simulink model "AttitudeControl_ADRC_Sim"  (R2017b)
settings: Solver=ode4  StartTime=0.0  StopTime=2  FixedStep=0.004  RelTol=1e-3
StartFcn:
  | Init_control_adrc
values from neighbouring files (symbols this model uses):
  DEG2RAD = 0.0174533    [Init_control_adrc.m]
  DisturbOn = 0    [Init_control_adrc.m]
  Kd_YAW_AngleRate = 0.00    (= 0)    [Init_control_adrc.m]
  Ki_YAW_AngleRate = 0.01    [Init_control_adrc.m]
  Kp_YAW_AngleRate = 0.5    [Init_control_adrc.m]
  MAX_CONTROL_ANGLE_PITCH = 35    [Init_control_adrc.m]
  MAX_CONTROL_ANGLE_RATE_Y = 200    [Init_control_adrc.m]
  MAX_CONTROL_ANGLE_ROLL = 35    [Init_control_adrc.m]
  ModelInit_AngEuler = [0, 0, 0]    [Init_control_adrc.m]
  ModelInit_PosE = [0, 0, 0]    [Init_control_adrc.m]
  ModelInit_Rads = 0    [Init_control_adrc.m]
  ModelInit_RateB = [0, 0, 0]    [Init_control_adrc.m]
  ModelInit_VelB = [0, 0, 0]    [Init_control_adrc.m]
  Saturation_I_Y_Max = 0.2    [Init_control_adrc.m]
  Saturation_I_Y_Min = -0.2    [Init_control_adrc.m]
  SL_ESO_B0 = single(47.4)    [Init_control_adrc.m]
  SL_ESO_B01 = single(250.0)    [Init_control_adrc.m]
  SL_ESO_B02 = single(2000.0)    [Init_control_adrc.m]
  SL_ESO_B03 = single(3000.0)    [Init_control_adrc.m]
  SL_ESO_D = single(0.01)    [Init_control_adrc.m]
  SL_ESO_H = single(1.0)    [Init_control_adrc.m]
  SL_NLSEF_C = single(5.0)    [Init_control_adrc.m]
  SL_NLSEF_H = single(25.0)    [Init_control_adrc.m]
  SL_NLSEF_R = single(200.0)    [Init_control_adrc.m]
  SL_TD_H = single(1.0)    [Init_control_adrc.m]
  SL_TD_R = single(20.0)    [Init_control_adrc.m]
  tau2sigma = single(0.108)    [Init_control_adrc.m]
  THR_HOVER = 0.609    [Init_control_adrc.m]
undefined symbols (not defined in the file or in its folder): DiscIntNeverNeededParam, earthRadius, ModelParam_envGravityAcc, ModelParam_motorCr, ModelParam_motorJm, ModelParam_motorT, ModelParam_motorWb, ModelParam_rotorCm, ModelParam_rotorCt, ModelParam_uavCCm, ModelParam_uavCd, ModelParam_uavJ, ModelParam_uavMass, ModelParam_uavR, Receive, Send
libraries: aerolibfltsims x3, simulink x2, sharedutil x2, aerolibwind2 x1, aerolibanimutils x1
settings Model: Creator=wsh  LastModifiedBy=Mr Wang
settings DebuggingCC: BusObjectLabelMismatch=error
settings CodeAppCC: StateflowObjectComments=on

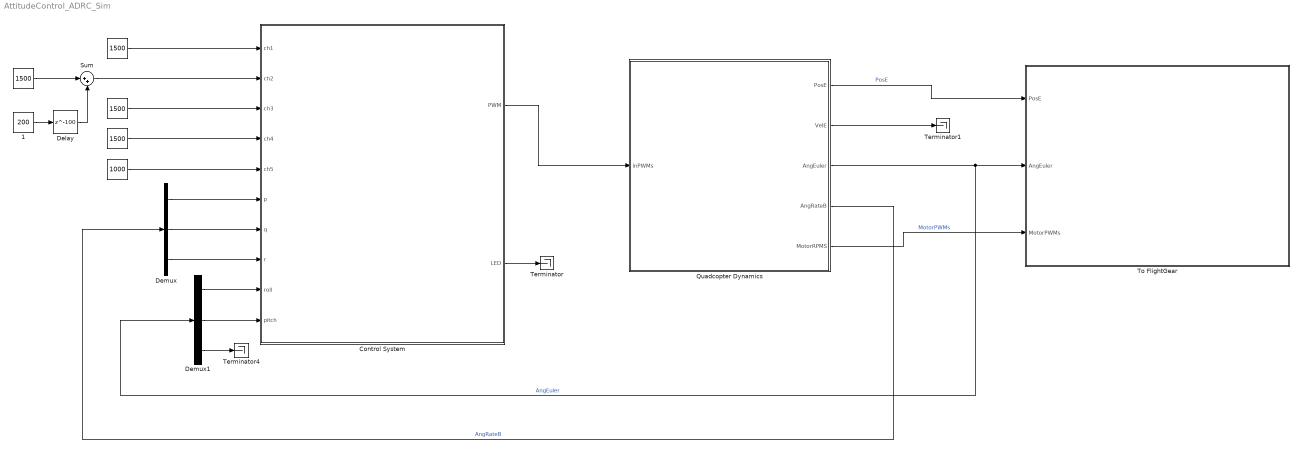
== system AttitudeControl_ADRC_Sim ==
  " " : Constant  Value=1000  OutDataTypeStr=uint16
  "  " : Constant  Value=1500  OutDataTypeStr=uint16
  "   " : Constant  Value=1500  OutDataTypeStr=uint16
  "      " : Constant  Value=1500  OutDataTypeStr=uint16
  "          " : Constant  Value=1500  OutDataTypeStr=uint16
  "  1" : Constant  Value=200  OutDataTypeStr=uint16
  Control System : Subsystem
      mask Display: image('icon\pixhawk.png');
  Delay : Delay  DelayLength=100  InitialCondition=0
  Demux : Demux  Outputs=3
  Demux1 : Demux  Outputs=3
  Quadcopter Dynamics : Subsystem
      mask Display: image('./icon/F450.png');
  Sum : Sum  Inputs=|++
  Terminator : Terminator
  Terminator1 : Terminator
  Terminator4 : Terminator
  To FlightGear : Subsystem
      mask Display: image('./icon/FlightGear.png');
  wires:
  Quadcopter Dynamics/1(PosE) -> To FlightGear/1(PosE)  "PosE"
  Quadcopter Dynamics/5(MotorRPMS) -> To FlightGear/3(MotorPWMs)  "MotorPWMs"
  Control System/2(LED) -> Terminator/1
  Quadcopter Dynamics/3(AngEuler) -> Demux1/1, To FlightGear/2(AngEuler)  "AngEuler"
  Quadcopter Dynamics/4(AngRateB) -> Demux/1  "AngRateB"
  Demux/1 -> Control System/6(p)
  Demux/2 -> Control System/7(q)
  Demux/3 -> Control System/8(r)
  Demux1/1 -> Control System/9(roll)
  Demux1/2 -> Control System/10(pitch)
  Demux1/3 -> Terminator4/1
  Quadcopter Dynamics/2(VelE) -> Terminator1/1
  Control System/1(PWM) -> Quadcopter Dynamics/1(inPWMs)
  Delay/1 -> Sum/2
  "  1"/1 -> Delay/1
  "  "/1 -> Sum/1
  " "/1 -> Control System/5(ch5)
  "      "/1 -> Control System/3(ch3)
  "          "/1 -> Control System/4(ch4)
  "   "/1 -> Control System/1(ch1)
  Sum/1 -> Control System/2(ch2)

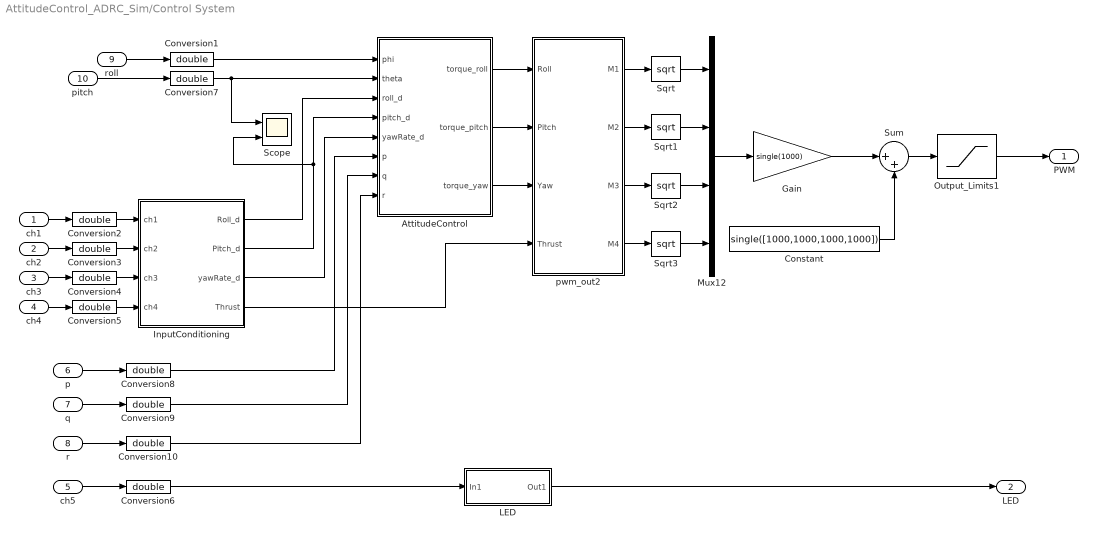
== system AttitudeControl_ADRC_Sim/Control System ==
  ch1 : Inport  OutDataTypeStr=uint16  PortDimensions=1
  ch2 : Inport  Port=2  OutDataTypeStr=uint16  PortDimensions=1
  ch3 : Inport  Port=3  OutDataTypeStr=uint16  PortDimensions=1
  ch4 : Inport  Port=4  OutDataTypeStr=uint16  PortDimensions=1
  ch5 : Inport  Port=5  OutDataTypeStr=uint16  PortDimensions=1  Interpolate=off
  p : Inport  Port=6  PortDimensions=1
  q : Inport  Port=7  PortDimensions=1
  r : Inport  Port=8  PortDimensions=1
  roll : Inport  Port=9  PortDimensions=1
  pitch : Inport  Port=10  PortDimensions=1
  AttitudeControl : Subsystem
  Constant : Constant  Value=single([1000,1000,1000,1000])
  Conversion{1..10} (10 alike) : DataTypeConversion  OutDataTypeStr=double
  Gain : Gain  Gain=single(1000)
  InputConditioning : Subsystem
  "LED " : Subsystem
  Mux12 : Mux
  Output_Limits1 : Saturate  Priority=2  UpperLimit=2000  LowerLimit=1000
  Scope : Scope  NumInputPorts=2
  Sqrt{,1..3} (4 alike) : Sqrt  SaturateOnIntegerOverflow=on
  Sum : Sum  Inputs=|++
  pwm_out2 : MATLAB Function  SystemSampleTime=0.004
  PWM : Outport
  LED : Outport  Port=2  PortDimensions=1
  wires:
  Mux12/1 -> Gain/1
  AttitudeControl/2(torque_pitch) -> pwm_out2/2(Pitch)
  AttitudeControl/1(torque_roll) -> pwm_out2/1(Roll)
  ch3/1 -> Conversion4/1
  ch5/1 -> Conversion6/1
  pwm_out2/3(M3) -> Sqrt2/1
  pwm_out2/2(M2) -> Sqrt1/1
  r/1 -> Conversion10/1
  AttitudeControl/3(torque_yaw) -> pwm_out2/3(Yaw)
  q/1 -> Conversion9/1
  InputConditioning/3(yawRate_d) -> AttitudeControl/5(yawRate_d)
  p/1 -> Conversion8/1
  ch4/1 -> Conversion5/1
  pwm_out2/4(M4) -> Sqrt3/1
  "LED "/1(Out1) -> LED/1
  Conversion6/1 -> "LED "/1(In1)
  Conversion5/1 -> InputConditioning/4(ch4)
  Conversion4/1 -> InputConditioning/3(ch3)
  pitch/1 -> Conversion7/1
  roll/1 -> Conversion1/1
  ch1/1 -> Conversion2/1
  ch2/1 -> Conversion3/1
  Conversion1/1 -> AttitudeControl/1(phi)
  Conversion7/1 -> AttitudeControl/2(theta), Scope/1
  Conversion8/1 -> AttitudeControl/6(p)
  Conversion9/1 -> AttitudeControl/7(q)
  Conversion10/1 -> AttitudeControl/8(r)
  InputConditioning/4(Thrust) -> pwm_out2/4(Thrust)
  Conversion2/1 -> InputConditioning/1("ch1 ")
  Conversion3/1 -> InputConditioning/2(ch2)
  InputConditioning/1(Roll_d) -> AttitudeControl/3(roll_d)
  InputConditioning/2(Pitch_d) -> Scope/2, AttitudeControl/4(pitch_d)
  pwm_out2/1(M1) -> Sqrt/1
  Sqrt/1 -> Mux12/1
  Sqrt1/1 -> Mux12/2
  Sqrt2/1 -> Mux12/3
  Sqrt3/1 -> Mux12/4
  Gain/1 -> Sum/1
  Constant/1 -> Sum/2
  Sum/1 -> Output_Limits1/1
  Output_Limits1/1 -> PWM/1

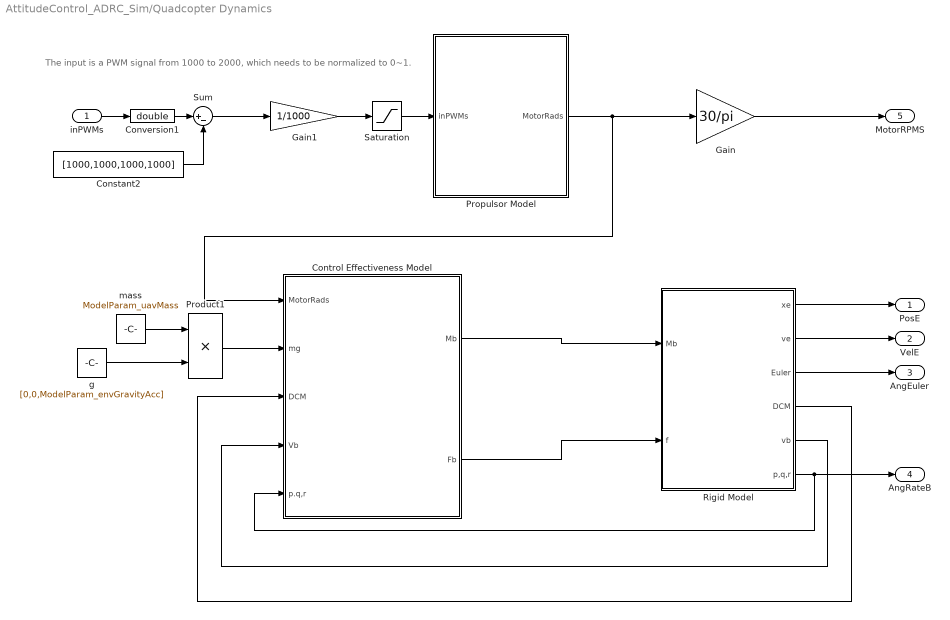
== system AttitudeControl_ADRC_Sim/Quadcopter Dynamics ==
  note: The input is a PWM signal from 1000 to 2000,
      | which needs to be normalized to 0~1.
  inPWMs : Inport
  Constant2 : Constant  Value=[1000,1000,1000,1000]
  Control Effectiveness Model : Subsystem
  Conversion1 : DataTypeConversion  OutDataTypeStr=double
  Gain : Gain  Gain=30/pi
  Gain1 : Gain  Gain=1/1000
  Product1 : Product
  Propulsor Model : Subsystem
  Rigid Model : Subsystem
  Saturation : Saturate  UpperLimit=1  LowerLimit=0
  Sum : Sum  Inputs=|+-
  g : Constant  Value=[0,0,ModelParam_envGravityAcc]
  mass : Constant  Value=ModelParam_uavMass
  PosE : Outport
  VelE : Outport  Port=2
  AngEuler : Outport  Port=3
  AngRateB : Outport  Port=4
  MotorRPMS : Outport  Port=5
  wires:
  Saturation/1 -> Propulsor Model/1(inPWMs)
  Rigid Model/6("p,q,r ") -> Control Effectiveness Model/5(p.q,r), AngRateB/1
  mass/1 -> Product1/1
  Rigid Model/4(DCM) -> Control Effectiveness Model/3(DCM)
  Propulsor Model/1(MotorRads) -> Gain/1, Control Effectiveness Model/1(MotorRads)
  Gain1/1 -> Saturation/1
  Rigid Model/2(ve) -> VelE/1
  Sum/1 -> Gain1/1
  Product1/1 -> Control Effectiveness Model/2(mg)
  Rigid Model/5("vb ") -> Control Effectiveness Model/4(Vb)
  Rigid Model/1("xe ") -> PosE/1
  Rigid Model/3(Euler) -> AngEuler/1
  Control Effectiveness Model/1(Mb) -> Rigid Model/1(Mb)
  inPWMs/1 -> Conversion1/1
  Control Effectiveness Model/2(Fb) -> Rigid Model/2(f)
  Constant2/1 -> Sum/2
  g/1 -> Product1/2
  Gain/1 -> MotorRPMS/1
  Conversion1/1 -> Sum/1

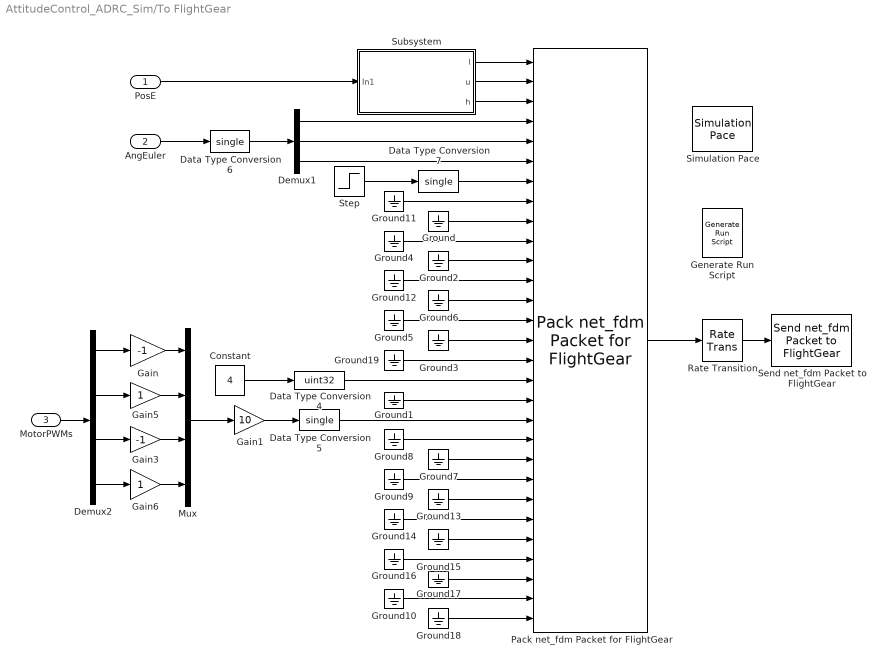
== system AttitudeControl_ADRC_Sim/To FlightGear ==
  PosE : Inport
  AngEuler : Inport  Port=2
  MotorPWMs : Inport  Port=3
  Constant : Constant  Value=4
  Data Type Conversion4 : DataTypeConversion  OutDataTypeStr=uint32
  Data Type Conversion5 : DataTypeConversion  OutDataTypeStr=single
  Data Type Conversion6 : DataTypeConversion  OutDataTypeStr=single
  Data Type Conversion7 : DataTypeConversion  OutDataTypeStr=single
  Demux1 : Demux  Outputs=3
  Demux2 : Demux
  Gain : Gain  Gain=-1
  Gain1 : Gain  Gain=10
  Gain3 : Gain  Gain=-1
  Gain5 : Gain
  Gain6 : Gain
  Generate Run Script : aerolibfltsims/Generate Run Script  OutputFileName=runfg_myownUAV.bat  FlightGearBaseDirectory=C:\Program Files\FlightGear 2016.1.2  GeometryModelName=myownUAV  DestinationPort=5502  OriginAddress=127.0.0.1  OriginPort=5505  LocalAddress=127.0.0.1  AirportId=KSFO  RunwayId=10L  InitialAltitude=0  InitialHeading=0  OffsetDistance=0  OffsetAzimuth=0  GenerateFile=off  Architecture=Default  dataFlow=Send-Receive
  Ground{,1..19} (20 alike) : Ground
  Mux : Mux
  Pack net_fdm Packet for FlightGear : aerolibfltsims/Pack net_fdm Packet for FlightGear  FlightGearVersion=v2016.1  ShowPositionAttitudeInputs=on  ShowVelocityAccelerationInputs=off  ShowControlSurfacePositionInputs=on  ShowEngineFuelInputs=on  ShowLandingGearInputs=off  ShowEnvironmentInputs=off  SampleTime=0.04
      settings: SourceProductName=Aerospace Blockset  SourceProductBaseCode=AE
  Rate Transition : RateTransition
  Send net_fdm Packet to FlightGear : aerolibfltsims/Send net_fdm Packet to FlightGear  DestinationIpAddress=127.0.0.1  DestinationPort=5502  LocalIpPort=-1  varLen=off  SampleTime=0.04
      settings: SourceProductName=Aerospace Blockset  SourceProductBaseCode=AE
  Simulation Pace : aerolibanimutils/Simulation Pace  SimulationPace=1  SleepMode=MATLAB Thread  OutputPaceError=off  SampleTime=-1
      settings: AttributesFormatString=%<SimulationPace> sec/sec
  Step : Step  Time=0  SampleTime=0
  Subsystem : Subsystem
  wires:
  Pack net_fdm Packet for FlightGear/1 -> Rate Transition/1
  Data Type Conversion7/1 -> Pack net_fdm Packet for FlightGear/7
  Ground8/1 -> Pack net_fdm Packet for FlightGear/20
  Ground/1 -> Pack net_fdm Packet for FlightGear/9
  Ground7/1 -> Pack net_fdm Packet for FlightGear/21
  Ground9/1 -> Pack net_fdm Packet for FlightGear/22
  Ground13/1 -> Pack net_fdm Packet for FlightGear/23
  Ground14/1 -> Pack net_fdm Packet for FlightGear/24
  Ground15/1 -> Pack net_fdm Packet for FlightGear/25
  Ground16/1 -> Pack net_fdm Packet for FlightGear/26
  Ground17/1 -> Pack net_fdm Packet for FlightGear/27
  Ground10/1 -> Pack net_fdm Packet for FlightGear/28
  Ground18/1 -> Pack net_fdm Packet for FlightGear/29
  Step/1 -> Data Type Conversion7/1
  Data Type Conversion4/1 -> Pack net_fdm Packet for FlightGear/17
  Ground1/1 -> Pack net_fdm Packet for FlightGear/18
  Ground3/1 -> Pack net_fdm Packet for FlightGear/15
  Ground5/1 -> Pack net_fdm Packet for FlightGear/14
  Ground6/1 -> Pack net_fdm Packet for FlightGear/13
  Ground4/1 -> Pack net_fdm Packet for FlightGear/10
  Ground11/1 -> Pack net_fdm Packet for FlightGear/8
  Constant/1 -> Data Type Conversion4/1
  Data Type Conversion5/1 -> Pack net_fdm Packet for FlightGear/19
  Ground2/1 -> Pack net_fdm Packet for FlightGear/11
  Ground12/1 -> Pack net_fdm Packet for FlightGear/12
  AngEuler/1 -> Data Type Conversion6/1
  MotorPWMs/1 -> Demux2/1
  Mux/1 -> Gain1/1
  Demux2/1 -> Gain/1
  Demux2/3 -> Gain3/1
  Gain/1 -> Mux/1
  Gain3/1 -> Mux/3
  Demux2/2 -> Gain5/1
  Gain5/1 -> Mux/2
  Demux2/4 -> Gain6/1
  Gain6/1 -> Mux/4
  Rate Transition/1 -> Send net_fdm Packet to FlightGear/1
  PosE/1 -> Subsystem/1(In1)
  Subsystem/1("l ") -> Pack net_fdm Packet for FlightGear/1
  Subsystem/2(u) -> Pack net_fdm Packet for FlightGear/2
  Subsystem/3(h) -> Pack net_fdm Packet for FlightGear/3
  Ground19/1 -> Pack net_fdm Packet for FlightGear/16
  Demux1/1 -> Pack net_fdm Packet for FlightGear/4
  Demux1/2 -> Pack net_fdm Packet for FlightGear/5
  Demux1/3 -> Pack net_fdm Packet for FlightGear/6
  Data Type Conversion6/1 -> Demux1/1
  Gain1/1 -> Data Type Conversion5/1

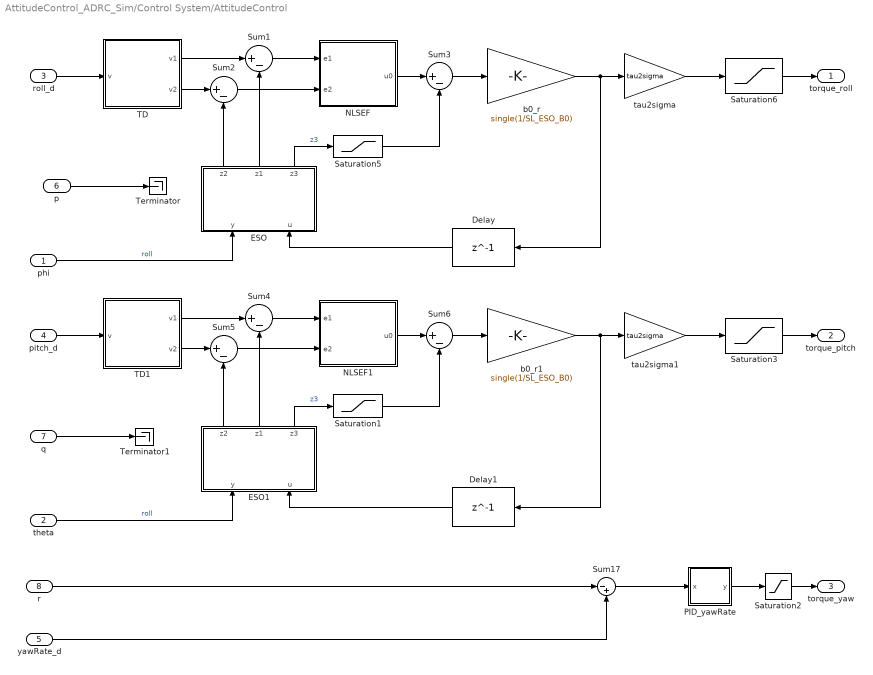
== system AttitudeControl_ADRC_Sim/Control System/AttitudeControl ==
  phi : Inport
  theta : Inport  Port=2
  roll_d : Inport  Port=3
  pitch_d : Inport  Port=4
  yawRate_d : Inport  Port=5
  p : Inport  Port=6
  q : Inport  Port=7
  r : Inport  Port=8
  Delay : Delay  DelayLength=1  InitialCondition=0
  Delay1 : Delay  DelayLength=1  InitialCondition=0
  ESO : Subsystem
  ESO1 : Subsystem
  NLSEF : Subsystem
  NLSEF1 : Subsystem
  PID_yawRate : Subsystem
  Saturation1 : Saturate  UpperLimit=SL_NLSEF_R*0.5  LowerLimit=-SL_NLSEF_R*0.5
  Saturation2 : Saturate
  Saturation3 : Saturate  UpperLimit=0.4  LowerLimit=-0.4
  Saturation5 : Saturate  UpperLimit=SL_NLSEF_R*0.5  LowerLimit=-SL_NLSEF_R*0.5
  Saturation6 : Saturate  UpperLimit=0.4  LowerLimit=-0.4
  Sum{1..6} (6 alike) : Sum  Inputs=|+-
  Sum17 : Sum  Inputs=|-+
  TD : Subsystem
  TD1 : Subsystem
  Terminator : Terminator
  Terminator1 : Terminator
  b0_r : Gain  Gain=single(1/SL_ESO_B0)
  b0_r1 : Gain  Gain=single(1/SL_ESO_B0)
  tau2sigma : Gain  Gain=tau2sigma
  tau2sigma1 : Gain  Gain=tau2sigma
  torque_roll : Outport
  torque_pitch : Outport  Port=2
  torque_yaw : Outport  Port=3
  wires:
  r/1 -> Sum17/1
  Sum17/1 -> PID_yawRate/1(x)
  PID_yawRate/1(y) -> Saturation2/1
  yawRate_d/1 -> Sum17/2
  Saturation2/1 -> torque_yaw/1
  ESO/1(z2) -> Sum2/2
  ESO/3(z3) -> Saturation5/1  "z3"
  roll_d/1 -> TD/1(v)
  ESO/2(z1) -> Sum1/2
  Saturation5/1 -> Sum3/2
  Sum3/1 -> b0_r/1
  TD/1(v1) -> Sum1/1
  Delay/1 -> ESO/2(u)
  tau2sigma/1 -> Saturation6/1
  b0_r/1 -> tau2sigma/1, Delay/1
  Sum1/1 -> NLSEF/1(e1)
  phi/1 -> ESO/1(y)  "roll"
  NLSEF/1(u0) -> Sum3/1
  Saturation6/1 -> torque_roll/1
  TD/2(v2) -> Sum2/1
  Sum2/1 -> NLSEF/2(e2)
  theta/1 -> ESO1/1(y)  "roll"
  pitch_d/1 -> TD1/1(v)
  Sum5/1 -> NLSEF1/2(e2)
  TD1/2(v2) -> Sum5/1
  NLSEF1/1(u0) -> Sum6/1
  Delay1/1 -> ESO1/2(u)
  Saturation3/1 -> torque_pitch/1
  b0_r1/1 -> tau2sigma1/1, Delay1/1
  TD1/1(v1) -> Sum4/1
  tau2sigma1/1 -> Saturation3/1
  Sum4/1 -> NLSEF1/1(e1)
  ESO1/3(z3) -> Saturation1/1  "z3"
  Saturation1/1 -> Sum6/2
  ESO1/2(z1) -> Sum4/2
  ESO1/1(z2) -> Sum5/2
  Sum6/1 -> b0_r1/1
  p/1 -> Terminator/1
  q/1 -> Terminator1/1

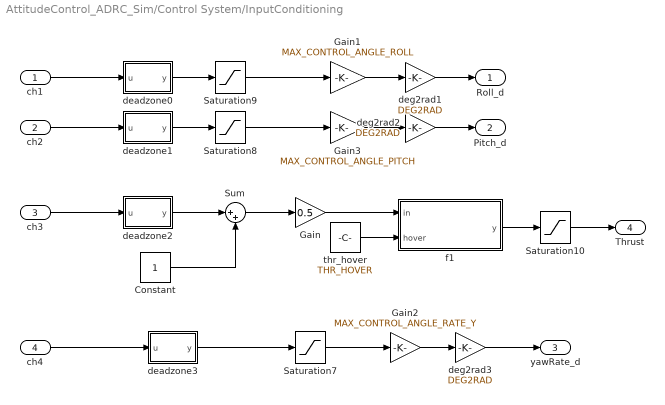
== system AttitudeControl_ADRC_Sim/Control System/InputConditioning ==
  "ch1 " : Inport
  ch2 : Inport  Port=2
  ch3 : Inport  Port=3
  ch4 : Inport  Port=4
  Constant : Constant
  Gain : Gain  Gain=0.5
  Gain1 : Gain  Gain=MAX_CONTROL_ANGLE_ROLL  OutDataTypeStr=Inherit: Inherit via back propagation
  Gain2 : Gain  Gain=MAX_CONTROL_ANGLE_RATE_Y
  Gain3 : Gain  Gain=MAX_CONTROL_ANGLE_PITCH  OutDataTypeStr=Inherit: Inherit via back propagation
  Saturation10 : Saturate  UpperLimit=1  LowerLimit=0
  Saturation7 : Saturate  UpperLimit=1  LowerLimit=-1
  Saturation8 : Saturate  UpperLimit=1  LowerLimit=-1
  Saturation9 : Saturate  UpperLimit=1  LowerLimit=-1
  Sum : Sum  Inputs=|++
  deadzone0 : MATLAB Function  TreatAsAtomicUnit=on
  deadzone1 : MATLAB Function  TreatAsAtomicUnit=on
  deadzone2 : MATLAB Function  TreatAsAtomicUnit=on
  deadzone3 : MATLAB Function  TreatAsAtomicUnit=on
  deg2rad1 : Gain  Gain=DEG2RAD
  deg2rad2 : Gain  Gain=DEG2RAD
  deg2rad3 : Gain  Gain=DEG2RAD
  f1 : MATLAB Function  TreatAsAtomicUnit=on
  "thr_hover " : Constant  Value=THR_HOVER
  Roll_d : Outport
  Pitch_d : Outport  Port=2
  yawRate_d : Outport  Port=3
  Thrust : Outport  Port=4
  wires:
  deadzone2/1(y) -> Sum/1
  ch3/1 -> deadzone2/1(u)
  deadzone1/1(y) -> Saturation8/1
  Saturation10/1 -> Thrust/1
  deadzone0/1(y) -> Saturation9/1
  "ch1 "/1 -> deadzone0/1(u)
  ch2/1 -> deadzone1/1(u)
  Saturation9/1 -> Gain1/1
  Saturation8/1 -> Gain3/1
  Gain3/1 -> deg2rad2/1
  Constant/1 -> Sum/2
  Sum/1 -> Gain/1
  Gain1/1 -> deg2rad1/1
  deg2rad1/1 -> Roll_d/1
  deg2rad2/1 -> Pitch_d/1
  Saturation7/1 -> Gain2/1
  deadzone3/1(y) -> Saturation7/1
  ch4/1 -> deadzone3/1(u)
  Gain2/1 -> deg2rad3/1
  deg2rad3/1 -> yawRate_d/1
  "thr_hover "/1 -> f1/2(hover)
  Gain/1 -> f1/1(in)
  f1/1(y) -> Saturation10/1

== system AttitudeControl_ADRC_Sim/Control System/LED  ==
  In1 : Inport
  Compare To Constant3 : simulink/Logic and Bit Operations/Compare To Constant  relop=>=  const=uint16(1500)  OutDataTypeStr=boolean
  Out1 : Outport
  wires:
  Compare To Constant3/1 -> Out1/1
  In1/1 -> Compare To Constant3/1

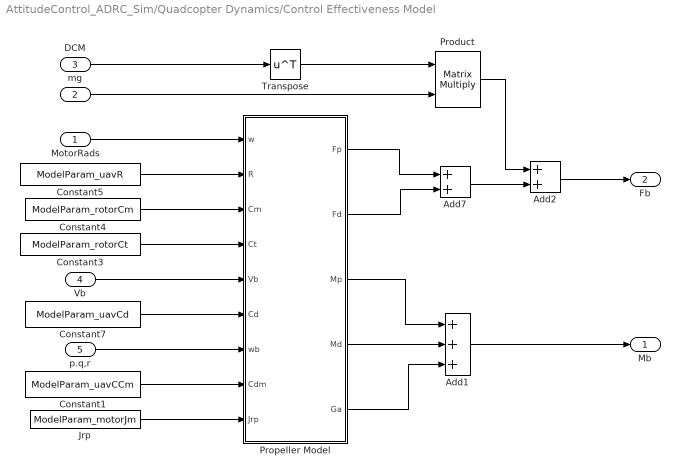
== system AttitudeControl_ADRC_Sim/Quadcopter Dynamics/Control Effectiveness Model ==
  MotorRads : Inport
  mg : Inport  Port=2
  DCM : Inport  Port=3
  Vb : Inport  Port=4
  p.q,r : Inport  Port=5
  Add1 : Sum  Inputs=+++
  Add2 : Sum
  Add7 : Sum
  Constant1 : Constant  Value=ModelParam_uavCCm
  Constant3 : Constant  Value=ModelParam_rotorCt
  Constant4 : Constant  Value=ModelParam_rotorCm
  Constant5 : Constant  Value=ModelParam_uavR
  Constant7 : Constant  Value=ModelParam_uavCd
  Jrp : Constant  Value=ModelParam_motorJm
  Product : Product  Multiplication=Matrix(*)
  Propeller Model : MATLAB Function  TreatAsAtomicUnit=on
  Transpose : Math  Operator=transpose  SaturateOnIntegerOverflow=on
  Mb : Outport
  Fb : Outport  Port=2
  wires:
  Add2/1 -> Fb/1
  Constant3/1 -> Propeller Model/4(Ct)
  Propeller Model/2(Fd) -> Add7/2
  Add7/1 -> Add2/2
  Propeller Model/1(Fp) -> Add7/1
  Product/1 -> Add2/1
  mg/1 -> Product/2
  DCM/1 -> Transpose/1
  Constant7/1 -> Propeller Model/6(Cd)
  Vb/1 -> Propeller Model/5(Vb)
  Constant5/1 -> Propeller Model/2(R)
  Constant4/1 -> Propeller Model/3(Cm)
  MotorRads/1 -> Propeller Model/1(w)
  Transpose/1 -> Product/1
  Propeller Model/3(Mp) -> Add1/1
  Propeller Model/4(Md) -> Add1/2
  Add1/1 -> Mb/1
  p.q,r/1 -> Propeller Model/7(wb)
  Constant1/1 -> Propeller Model/8(Cdm)
  Jrp/1 -> Propeller Model/9(Jrp)
  Propeller Model/5(Ga) -> Add1/3

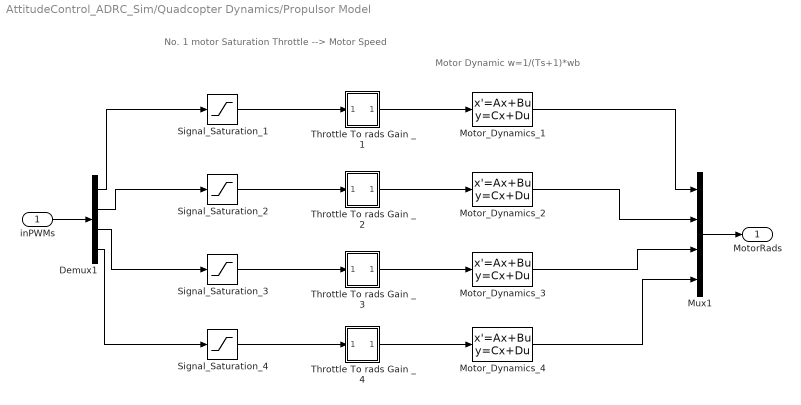
== system AttitudeControl_ADRC_Sim/Quadcopter Dynamics/Propulsor Model ==
  note: Motor Dynamic
      | w=1/(Ts+1)*wb
  note: No. 1 motor
      |
      |          Saturation             Throttle --> Motor Speed
  inPWMs : Inport
  Demux1 : Demux
  Motor_Dynamics_{1..4} (4 alike) : StateSpace  A=-1/ModelParam_motorT  C=1/ModelParam_motorT  D=0  InitialCondition=ModelInit_Rads*ModelParam_motorT
  Mux1 : Mux
  Signal_Saturation_{1..4} (4 alike) : Saturate  UpperLimit=1  LowerLimit=0
  Throttle To rads Gain _1 : Subsystem
  Throttle To rads Gain _2 : Subsystem
  Throttle To rads Gain _3 : Subsystem
  Throttle To rads Gain _4 : Subsystem
  MotorRads : Outport
  wires:
  Throttle To rads Gain _4/1(Out5) -> Motor_Dynamics_4/1
  Signal_Saturation_4/1 -> Throttle To rads Gain _4/1(In5)
  Signal_Saturation_3/1 -> Throttle To rads Gain _3/1(In5)
  Signal_Saturation_2/1 -> Throttle To rads Gain _2/1(In5)
  Motor_Dynamics_4/1 -> Mux1/4
  Motor_Dynamics_3/1 -> Mux1/3
  Motor_Dynamics_2/1 -> Mux1/2
  Motor_Dynamics_1/1 -> Mux1/1
  Signal_Saturation_1/1 -> Throttle To rads Gain _1/1(In5)
  Mux1/1 -> MotorRads/1
  Throttle To rads Gain _3/1(Out5) -> Motor_Dynamics_3/1
  Throttle To rads Gain _2/1(Out5) -> Motor_Dynamics_2/1
  Throttle To rads Gain _1/1(Out5) -> Motor_Dynamics_1/1
  inPWMs/1 -> Demux1/1
  Demux1/4 -> Signal_Saturation_4/1
  Demux1/3 -> Signal_Saturation_3/1
  Demux1/2 -> Signal_Saturation_2/1
  Demux1/1 -> Signal_Saturation_1/1

== system AttitudeControl_ADRC_Sim/Quadcopter Dynamics/Rigid Model ==
  Mb : Inport
  f : Inport  Port=2
  Rigid-Body Dynamic Model : Subsystem
  "Rigid-Body Kinematic Model " : Subsystem
  "xe " : Outport
  ve : Outport  Port=2
  Euler : Outport  Port=3
  DCM : Outport  Port=4
  "vb " : Outport  Port=5
  "p,q,r " : Outport  Port=6
  wires:
  Rigid-Body Dynamic Model/1("p,q,r ") -> "Rigid-Body Kinematic Model "/1(pqr), "p,q,r "/1
  "Rigid-Body Kinematic Model "/1(Euler) -> Euler/1
  "Rigid-Body Kinematic Model "/3(DCM) -> Rigid-Body Dynamic Model/3(DCM), DCM/1
  Mb/1 -> Rigid-Body Dynamic Model/1(Mb)
  f/1 -> Rigid-Body Dynamic Model/2(f)
  Rigid-Body Dynamic Model/2(ve) -> "Rigid-Body Kinematic Model "/2(ve), ve/1
  Rigid-Body Dynamic Model/3("vb ") -> "vb "/1
  "Rigid-Body Kinematic Model "/2("xe ") -> "xe "/1

== system AttitudeControl_ADRC_Sim/To FlightGear/Subsystem ==
  In1 : Inport
  Constant1 : Constant  Value=5  VectorParams1D=off
  Constant2 : Constant  Value=-2.1361  VectorParams1D=off
  Constant3 : Constant  Value=0.65673  VectorParams1D=off
  Demux : Demux  Outputs=3
  Gain1 : Gain  Gain=10/earthRadius
  Gain2 : Gain  Gain=10/earthRadius
  Gain4 : Gain
  Gain8 : Gain  Gain=-10
  Sum10 : Sum  Inputs=|++
  Sum8 : Sum  Inputs=|++
  Sum9 : Sum  Inputs=|++
  "l " : Outport
  u : Outport  Port=2
  h : Outport  Port=3
  wires:
  Constant3/1 -> Sum9/2
  Constant1/1 -> Sum10/2
  Demux/1 -> Gain4/1
  Demux/3 -> Gain8/1
  Constant2/1 -> Sum8/2
  Gain2/1 -> Sum9/1
  Gain1/1 -> Sum8/1
  Gain8/1 -> Sum10/1
  Demux/2 -> Gain1/1
  Gain4/1 -> Gain2/1
  Sum10/1 -> h/1
  Sum9/1 -> u/1
  In1/1 -> Demux/1
  Sum8/1 -> "l "/1

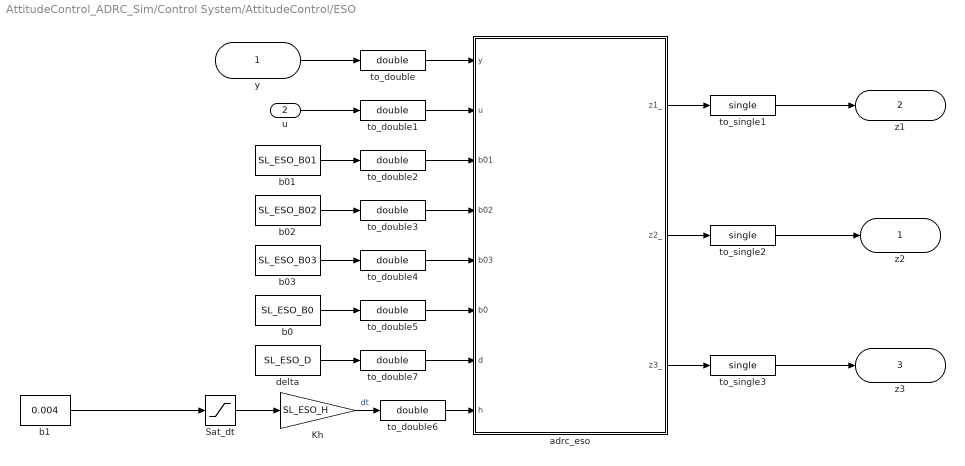
== system AttitudeControl_ADRC_Sim/Control System/AttitudeControl/ESO ==
  y : Inport
  u : Inport  Port=2
  Kh : Gain  Priority=4  Gain=SL_ESO_H
  Sat_dt : Saturate  UpperLimit=0.02  LowerLimit=0.004
  adrc_eso : MATLAB Function  TreatAsAtomicUnit=on
  b0 : Constant  Value=SL_ESO_B0
  b01 : Constant  Value=SL_ESO_B01
  b02 : Constant  Value=SL_ESO_B02
  b03 : Constant  Value=SL_ESO_B03
  b1 : Constant  Value=0.004
  delta : Constant  Value=SL_ESO_D
  to_double{,1..7} (8 alike) : DataTypeConversion  OutDataTypeStr=double
  to_single1 : DataTypeConversion  OutDataTypeStr=single
  to_single2 : DataTypeConversion  OutDataTypeStr=single
  to_single3 : DataTypeConversion  OutDataTypeStr=single
  z2 : Outport
  z1 : Outport  Port=2  OutDataTypeStr=single
  z3 : Outport  Port=3
  wires:
  y/1 -> to_double/1
  u/1 -> to_double1/1
  b1/1 -> Sat_dt/1
  Sat_dt/1 -> Kh/1
  Kh/1 -> to_double6/1  "dt"
  adrc_eso/1(z1_) -> to_single1/1
  adrc_eso/2(z2_) -> to_single2/1
  adrc_eso/3(z3_) -> to_single3/1
  b01/1 -> to_double2/1
  b02/1 -> to_double3/1
  b03/1 -> to_double4/1
  b0/1 -> to_double5/1
  to_double/1 -> adrc_eso/1(y)
  to_double1/1 -> adrc_eso/2(u)
  to_double2/1 -> adrc_eso/3(b01)
  to_double3/1 -> adrc_eso/4(b02)
  to_double4/1 -> adrc_eso/5(b03)
  to_double5/1 -> adrc_eso/6(b0)
  to_single1/1 -> z1/1
  to_single2/1 -> z2/1
  to_single3/1 -> z3/1
  to_double6/1 -> adrc_eso/8(h)
  delta/1 -> to_double7/1
  to_double7/1 -> adrc_eso/7(d)

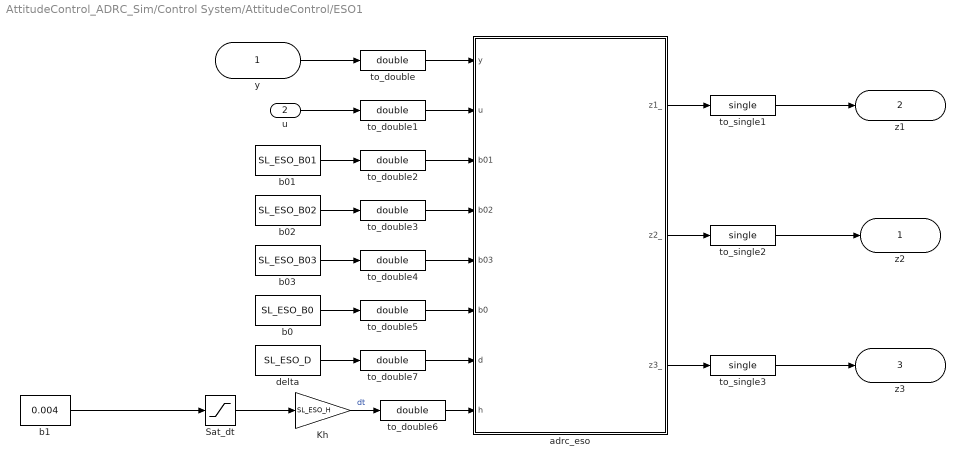
== system AttitudeControl_ADRC_Sim/Control System/AttitudeControl/ESO1 ==
  y : Inport
  u : Inport  Port=2
  Kh : Gain  Priority=4  Gain=SL_ESO_H
  Sat_dt : Saturate  UpperLimit=0.02  LowerLimit=0.004
  adrc_eso : MATLAB Function  TreatAsAtomicUnit=on
  b0 : Constant  Value=SL_ESO_B0
  b01 : Constant  Value=SL_ESO_B01
  b02 : Constant  Value=SL_ESO_B02
  b03 : Constant  Value=SL_ESO_B03
  b1 : Constant  Value=0.004
  delta : Constant  Value=SL_ESO_D
  to_double{,1..7} (8 alike) : DataTypeConversion  OutDataTypeStr=double
  to_single1 : DataTypeConversion  OutDataTypeStr=single
  to_single2 : DataTypeConversion  OutDataTypeStr=single
  to_single3 : DataTypeConversion  OutDataTypeStr=single
  z2 : Outport
  z1 : Outport  Port=2  OutDataTypeStr=single
  z3 : Outport  Port=3
  wires:
  y/1 -> to_double/1
  u/1 -> to_double1/1
  b1/1 -> Sat_dt/1
  Sat_dt/1 -> Kh/1
  Kh/1 -> to_double6/1  "dt"
  adrc_eso/1(z1_) -> to_single1/1
  adrc_eso/2(z2_) -> to_single2/1
  adrc_eso/3(z3_) -> to_single3/1
  b01/1 -> to_double2/1
  b02/1 -> to_double3/1
  b03/1 -> to_double4/1
  b0/1 -> to_double5/1
  to_double/1 -> adrc_eso/1(y)
  to_double1/1 -> adrc_eso/2(u)
  to_double2/1 -> adrc_eso/3(b01)
  to_double3/1 -> adrc_eso/4(b02)
  to_double4/1 -> adrc_eso/5(b03)
  to_double5/1 -> adrc_eso/6(b0)
  to_single1/1 -> z1/1
  to_single2/1 -> z2/1
  to_single3/1 -> z3/1
  to_double6/1 -> adrc_eso/8(h)
  delta/1 -> to_double7/1
  to_double7/1 -> adrc_eso/7(d)

== system AttitudeControl_ADRC_Sim/Control System/AttitudeControl/NLSEF ==
  note: u0 = -fhan(e1,ce2,r,h1)
  e1 : Inport
  e2 : Inport  Port=2
  Constant : Constant  Value=0.004  OutDataTypeStr=single
  Kh : Gain  Gain=SL_NLSEF_H
  Sat_dt : Saturate  UpperLimit=0.02  LowerLimit=0.004
  c : Gain  Gain=SL_NLSEF_C
  fhan : MATLAB Function  TreatAsAtomicUnit=on
  gain1 : Gain  Gain=-1
  r : Constant  Value=SL_NLSEF_R
  u0 : Outport
  wires:
  Kh/1 -> fhan/4(h)
  gain1/1 -> u0/1
  e1/1 -> fhan/1(x1)
  e2/1 -> c/1
  r/1 -> fhan/3(r)  "r"
  c/1 -> fhan/2(x2)
  Sat_dt/1 -> Kh/1
  fhan/1(y) -> gain1/1
  Constant/1 -> Sat_dt/1  "dt"

== system AttitudeControl_ADRC_Sim/Control System/AttitudeControl/NLSEF1 ==
  note: u0 = -fhan(e1,ce2,r,h1)
  e1 : Inport
  e2 : Inport  Port=2
  Constant : Constant  Value=0.004  OutDataTypeStr=single
  Kh : Gain  Gain=SL_NLSEF_H
  Sat_dt : Saturate  UpperLimit=0.02  LowerLimit=0.004
  c : Gain  Gain=SL_NLSEF_C
  fhan : MATLAB Function  TreatAsAtomicUnit=on
  gain1 : Gain  Gain=-1
  r : Constant  Value=SL_NLSEF_R
  u0 : Outport
  wires:
  Kh/1 -> fhan/4(h)
  gain1/1 -> u0/1
  e1/1 -> fhan/1(x1)
  e2/1 -> c/1
  r/1 -> fhan/3(r)  "r"
  c/1 -> fhan/2(x2)
  Sat_dt/1 -> Kh/1
  fhan/1(y) -> gain1/1
  Constant/1 -> Sat_dt/1  "dt"

== system AttitudeControl_ADRC_Sim/Control System/AttitudeControl/PID_yawRate ==
  x : Inport
  Derivative Gain : Gain  DisableCoverage=on  Gain=Kd_YAW_AngleRate  ParamMin=-100  ParamMax=100  OutMin=-100  OutMax=100
  Discrete Derivative : simulink/Discrete/Discrete Derivative  gainval=1.0  ICPrevScaledInput=0.0  OutMin=[]  OutMax=[]  OutDataType=fixdt(1, 16)  OutScaling=2^-10  DoSatur=off
  Discrete-Time Integrator : DiscreteIntegrator  InitialConditionSetting=State (most efficient)  SampleTime=-1  LimitOutput=on  UpperSaturationLimit=Saturation_I_Y_Max  LowerSaturationLimit=Saturation_I_Y_Min  ICPrevOutput=DiscIntNeverNeededParam  ICPrevScaledInput=DiscIntNeverNeededParam
  Gain : Gain  Gain=Kp_YAW_AngleRate
  Integral Gain : Gain  DisableCoverage=on  Gain=Ki_YAW_AngleRate
  Sum : Sum  Inputs=+++
  y : Outport  InitialOutput=0
  wires:
  x/1 -> Gain/1, Integral Gain/1, Derivative Gain/1
  Integral Gain/1 -> Discrete-Time Integrator/1
  Derivative Gain/1 -> Discrete Derivative/1
  Gain/1 -> Sum/1
  Sum/1 -> y/1
  Discrete Derivative/1 -> Sum/3
  Discrete-Time Integrator/1 -> Sum/2

== system AttitudeControl_ADRC_Sim/Control System/AttitudeControl/TD ==
  note: v1(k+1)=v1(k)+h*v2(k)
      | v2(k+1)=v2(k)+h*fhan()
  v : Inport
  Constant : Constant  Value=0.004
  Gain : Gain  Gain=SL_TD_H
  Sat_dt : Saturate  UpperLimit=0.02  LowerLimit=0.004
  TD : MATLAB Function  TreatAsAtomicUnit=on
  r : Constant  Value=SL_TD_R
  to_double1 : DataTypeConversion  OutDataTypeStr=double
  to_double2 : DataTypeConversion  OutDataTypeStr=double
  to_double3 : DataTypeConversion  OutDataTypeStr=double
  to_single1 : DataTypeConversion  OutDataTypeStr=single
  to_single2 : DataTypeConversion  OutDataTypeStr=single
  v1 : Outport
  v2 : Outport  Port=2
  wires:
  v/1 -> to_double1/1
  TD/1(v1_) -> to_single1/1
  r/1 -> to_double2/1
  TD/2(v2_) -> to_single2/1
  Sat_dt/1 -> Gain/1
  Gain/1 -> to_double3/1
  to_double1/1 -> TD/1(v)
  to_double2/1 -> TD/2(r)
  to_double3/1 -> TD/3(h)
  to_single1/1 -> v1/1
  to_single2/1 -> v2/1
  Constant/1 -> Sat_dt/1

== system AttitudeControl_ADRC_Sim/Control System/AttitudeControl/TD1 ==
  note: v1(k+1)=v1(k)+h*v2(k)
      | v2(k+1)=v2(k)+h*fhan()
  v : Inport
  Constant : Constant  Value=0.004
  Gain : Gain  Gain=SL_TD_H
  Sat_dt : Saturate  UpperLimit=0.02  LowerLimit=0.004
  TD : MATLAB Function  TreatAsAtomicUnit=on
  r : Constant  Value=SL_TD_R
  to_double1 : DataTypeConversion  OutDataTypeStr=double
  to_double2 : DataTypeConversion  OutDataTypeStr=double
  to_double3 : DataTypeConversion  OutDataTypeStr=double
  to_single1 : DataTypeConversion  OutDataTypeStr=single
  to_single2 : DataTypeConversion  OutDataTypeStr=single
  v1 : Outport
  v2 : Outport  Port=2
  wires:
  v/1 -> to_double1/1
  TD/1(v1_) -> to_single1/1
  r/1 -> to_double2/1
  TD/2(v2_) -> to_single2/1
  Sat_dt/1 -> Gain/1
  Gain/1 -> to_double3/1
  to_double1/1 -> TD/1(v)
  to_double2/1 -> TD/2(r)
  to_double3/1 -> TD/3(h)
  to_single1/1 -> v1/1
  to_single2/1 -> v2/1
  Constant/1 -> Sat_dt/1

== system AttitudeControl_ADRC_Sim/Quadcopter Dynamics/Propulsor Model/Throttle To rads Gain _1 ==
  In5 : Inport
  Constant : Constant  Value=ModelParam_motorWb
  Gain : Gain  Gain=ModelParam_motorCr
  Sum1 : Sum  Inputs=++|
  Out5 : Outport
  wires:
  Constant/1 -> Sum1/1
  Gain/1 -> Sum1/2
  In5/1 -> Gain/1
  Sum1/1 -> Out5/1

== system AttitudeControl_ADRC_Sim/Quadcopter Dynamics/Propulsor Model/Throttle To rads Gain _2 ==
  In5 : Inport
  Constant : Constant  Value=ModelParam_motorWb
  Gain : Gain  Gain=ModelParam_motorCr
  Sum1 : Sum  Inputs=++|
  Out5 : Outport
  wires:
  Sum1/1 -> Out5/1
  In5/1 -> Gain/1
  Gain/1 -> Sum1/2
  Constant/1 -> Sum1/1

== system AttitudeControl_ADRC_Sim/Quadcopter Dynamics/Propulsor Model/Throttle To rads Gain _3 ==
  In5 : Inport
  Constant : Constant  Value=ModelParam_motorWb
  Gain : Gain  Gain=ModelParam_motorCr
  Sum1 : Sum  Inputs=++|
  Out5 : Outport
  wires:
  Constant/1 -> Sum1/1
  Gain/1 -> Sum1/2
  In5/1 -> Gain/1
  Sum1/1 -> Out5/1

== system AttitudeControl_ADRC_Sim/Quadcopter Dynamics/Propulsor Model/Throttle To rads Gain _4 ==
  In5 : Inport
  Constant : Constant  Value=ModelParam_motorWb
  Gain : Gain  Gain=ModelParam_motorCr
  Sum1 : Sum  Inputs=++|
  Out5 : Outport
  wires:
  Sum1/1 -> Out5/1
  In5/1 -> Gain/1
  Gain/1 -> Sum1/2
  Constant/1 -> Sum1/1

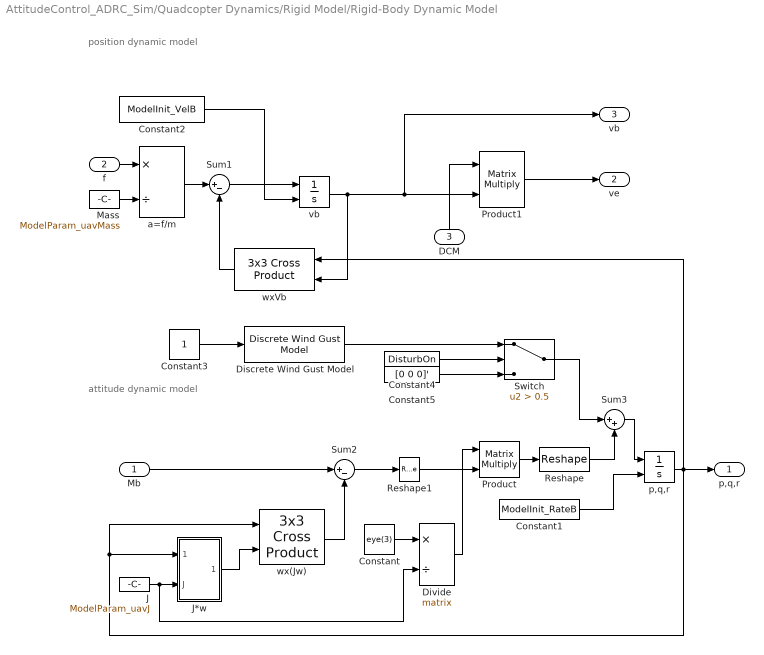
== system AttitudeControl_ADRC_Sim/Quadcopter Dynamics/Rigid Model/Rigid-Body Dynamic Model ==
  note: attitude dynamic model
  note: position dynamic model
  Mb : Inport
  f : Inport  Port=2
  DCM : Inport  Port=3
  " Mass " : Constant  Value=ModelParam_uavMass
  Constant : Constant  Value=eye(3)
  Constant1 : Constant  Value=ModelInit_RateB
  Constant2 : Constant  Value=ModelInit_VelB
  Constant3 : Constant
  Constant4 : Constant  Value=DisturbOn
  Constant5 : Constant  Value=[0 0 0]'
  Discrete Wind Gust Model : aerolibwind2/Discrete Wind Gust Model  units=Metric (MKS)  Gx=on  Gy=on  Gz=off  t_0=DisturbStartTime  d_m=[0.5 0.5 80]  v_m=[12 12 0]
      settings: SourceProductName=Aerospace Blockset
  Divide : Product  Inputs=*/  Multiplication=Matrix(*)
  "J " : Constant  Value=ModelParam_uavJ
  J*w : Subsystem
  Product : Product  Multiplication=Matrix(*)
  Product1 : Product  Multiplication=Matrix(*)
  Reshape : Reshape  OutputDimensionality=Customize  OutputDimensions=[3,1]
  Reshape1 : Reshape  OutputDimensionality=Column vector (2-D)
  Sum1 : Sum  Inputs=|+-
  Sum2 : Sum  Inputs=|+-
  Sum3 : Sum  Inputs=|++
  Switch : Switch  Criteria=u2 > Threshold  Threshold=0.5
  a=f/m : Product  Inputs=*/
  p,q,r : Integrator  InitialConditionSource=external
  vb : Integrator  InitialConditionSource=external
  wx(Jw) : sharedutil/3x3 Cross Product
      settings: SourceProductBaseCode=AE
  wxVb : sharedutil/3x3 Cross Product
      settings: SourceProductBaseCode=AE
  "p,q,r " : Outport
  ve : Outport  Port=2
  "vb " : Outport  Port=3
  wires:
  Product/1 -> Reshape/1
  Reshape1/1 -> Product/2
  Constant/1 -> Divide/1
  Divide/1 -> Product/1
  Sum2/1 -> Reshape1/1
  "J "/1 -> Divide/2, J*w/2(J)
  p,q,r/1 -> "p,q,r "/1, J*w/1(p q r), wx(Jw)/1, wxVb/1
  J*w/1("J*w ") -> wx(Jw)/2
  Mb/1 -> Sum2/1
  wx(Jw)/1 -> Sum2/2
  Constant2/1 -> vb/2
  f/1 -> a=f/m/1
  Product1/1 -> ve/1
  wxVb/1 -> Sum1/2
  a=f/m/1 -> Sum1/1
  Sum1/1 -> vb/1
  vb/1 -> Product1/2, "vb "/1, wxVb/2
  " Mass "/1 -> a=f/m/2
  DCM/1 -> Product1/1
  Reshape/1 -> Sum3/2
  Constant1/1 -> p,q,r/2
  Constant3/1 -> Discrete Wind Gust Model/1
  Discrete Wind Gust Model/1 -> Switch/1
  Sum3/1 -> p,q,r/1
  Constant4/1 -> Switch/2
  Constant5/1 -> Switch/3
  Switch/1 -> Sum3/1

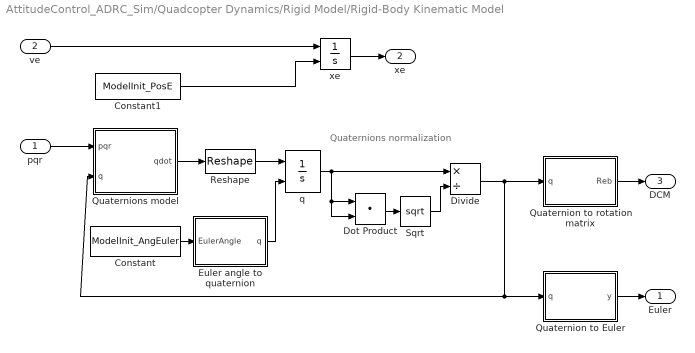
== system AttitudeControl_ADRC_Sim/Quadcopter Dynamics/Rigid Model/Rigid-Body Kinematic Model  ==
  note: Quaternions
      | normalization
  pqr : Inport
  ve : Inport  Port=2
  Constant : Constant  Value=ModelInit_AngEuler
  Constant1 : Constant  Value=ModelInit_PosE
  Divide : Product  Inputs=*/
  Dot Product : DotProduct  InputSameDT=on  OutDataTypeStr=Inherit: Inherit via internal rule
  Euler angle to quaternion : MATLAB Function
  Quaternion to Euler : MATLAB Function
  Quaternion to rotation matrix : MATLAB Function
  Quaternions model : MATLAB Function  TreatAsAtomicUnit=on
  Reshape : Reshape  OutputDimensionality=Customize  OutputDimensions=[4,1]
  Sqrt : Sqrt  SaturateOnIntegerOverflow=on
  q : Integrator  InitialConditionSource=external
  xe : Integrator  InitialConditionSource=external
  Euler : Outport
  "xe " : Outport  Port=2
  DCM : Outport  Port=3
  wires:
  Divide/1 -> Quaternion to rotation matrix/1(q), Quaternions model/2(q), Quaternion to Euler/1(q)
  Dot Product/1 -> Sqrt/1
  pqr/1 -> Quaternions model/1(pqr)
  q/1 -> Divide/1, Dot Product/1, Dot Product/2
  Quaternions model/1(qdot) -> Reshape/1
  Quaternion to rotation matrix/1(Reb) -> DCM/1
  Quaternion to Euler/1(y) -> Euler/1
  Constant/1 -> Euler angle to quaternion/1(EulerAngle)
  Euler angle to quaternion/1(q) -> q/2
  Reshape/1 -> q/1
  ve/1 -> xe/1
  xe/1 -> "xe "/1
  Constant1/1 -> xe/2
  Sqrt/1 -> Divide/2

== system AttitudeControl_ADRC_Sim/Quadcopter Dynamics/Rigid Model/Rigid-Body Dynamic Model/J*w ==
  p q r : Inport
  J : Inport  Port=2
  J*w : Product  Multiplication=Matrix(*)
  "J*w " : Outport
  wires:
  J*w/1 -> "J*w "/1
  J/1 -> J*w/1
  p q r/1 -> J*w/2

== matlab function AttitudeControl_ADRC_Sim/Control System/InputConditioning/deadzone0 ==
  data: u input; y output
function y = fcn(u)
%Function description:
%  Control the range of the remote control input from RCMin to RCMax, and set
%  a dead zone with a dead zone size of ±deadZone,the output y is
%  normalized to 0~1.You can get the RC calibration parameters in QGC.
RCMin = 1100;
RCMax = 1900;
RCMid = (RCMin + RCMax)/2;
deadZoneRate = 0.05;
deadZone = deadZoneRate*(RCMax - RCMin);
k = 1/(RCMax - RCMid - deadZone);
%Limiting
if(u < RCMin)
    u = RCMin;
elseif(u > RCMax)
    u = RCMax;
end
%dead zone and normalize
 if(u > RCMid + deadZone)
    y = (u-RCMid - deadZone)*k;
 elseif(u < RCMid - deadZone)
     y = (u - RCMid + deadZone)*k;
 else
     y = 0;
 end

 end

== matlab function AttitudeControl_ADRC_Sim/Control System/InputConditioning/deadzone1 ==
  data: u input; y output
function y = fcn(u)
%Function description:
%  Control the range of the remote control input from RCMin to RCMax, and set
%  a dead zone with a dead zone size of ±deadZone,the output y is
%  normalized to 0~1.You can get the RC calibration parameters in QGC.
RCMin = 1100;
RCMax = 1900;
RCMid = (RCMin + RCMax)/2;
deadZoneRate = 0.05;
deadZone = deadZoneRate*(RCMax - RCMin);
k = 1/(RCMax - RCMid - deadZone);
%Limiting
if(u < RCMin)
    u = RCMin;
elseif(u > RCMax)
    u = RCMax;
end
%dead zone and normalize
 if(u > RCMid + deadZone)
    y = (u-RCMid - deadZone)*k;
 elseif(u < RCMid - deadZone)
     y = (u - RCMid + deadZone)*k;
 else
     y = 0;
 end

 end

== matlab function AttitudeControl_ADRC_Sim/Control System/InputConditioning/deadzone2 ==
  data: u input; y output
function y = fcn(u)
%Function description:
%  Control the range of the remote control input from RCMin to RCMax, and set
%  a dead zone with a dead zone size of ±deadZone,the output y is
%  normalized to 0~1.You can get the RC calibration parameters in QGC.
RCMin = 1100;
RCMax = 1900;
RCMid = (RCMin + RCMax)/2;
deadZoneRate = 0.05;
deadZone = deadZoneRate*(RCMax - RCMin);
k = 1/(RCMax - RCMid - deadZone);
%Limiting
if(u < RCMin)
    u = RCMin;
elseif(u > RCMax)
    u = RCMax;
end
%dead zone and normalize
 if(u > RCMid + deadZone)
    y = (u-RCMid - deadZone)*k;
 elseif(u < RCMid - deadZone)
     y = (u - RCMid + deadZone)*k;
 else
     y = 0;
 end

 end

== matlab function AttitudeControl_ADRC_Sim/Control System/AttitudeControl/ESO1/adrc_eso ==
  settings: updateMethod=DISCRETE
  data: y input; u input; z1_ output; b01 input; b02 input; b03 input; b0 input; d input; h input; z2_ output; z3_ output
function [z1_, z2_, z3_] = adrc_eso(y, u, b01, b02, b03, b0, d, h)
persistent z1  z2 z3
if (isempty(z1) || isempty(z2) || isempty(z3))
    z1 = 0;
    z2 = 0;
    z3 = 0;
end
e = z1 - y;
fe = fal(e, 0.5, d);
fe1 = fal(e, 0.25, d);

z1_ = z1 + h*(z2 - b01*e);
z2_ = z2 + h*(z3 + b0*u - b02*fe);
z3_ = z3 - h*b03*fe1;

z1 = z1_;
z2 = z2_;
z3 = z3_;

end

function  y = fal( x, alpha, delta )

if abs(x) < delta
    y = x / delta^(1.0 - alpha);
else
    y = (abs(x)^alpha) * sign(x);
end

end

== matlab function AttitudeControl_ADRC_Sim/Control System/InputConditioning/deadzone3 ==
  data: u input; y output
function y = fcn(u)
%Function description:
%  Control the range of the remote control input from RCMin to RCMax, and set
%  a dead zone with a dead zone size of ±deadZone,the output y is
%  normalized to 0~1.You can get the RC calibration parameters in QGC.
RCMin = 1100;
RCMax = 1900;
RCMid = (RCMin + RCMax)/2;
deadZoneRate = 0.05;
deadZone = deadZoneRate*(RCMax - RCMin);
k = 1/(RCMax - RCMid - deadZone);
%Limiting
if(u < RCMin)
    u = RCMin;
elseif(u > RCMax)
    u = RCMax;
end
%dead zone and normalize
 if(u > RCMid + deadZone)
    y = (u-RCMid - deadZone)*k;
 elseif(u < RCMid - deadZone)
     y = (u - RCMid + deadZone)*k;
 else
     y = 0;
 end

 end

== matlab function AttitudeControl_ADRC_Sim/Control System/AttitudeControl/NLSEF1/fhan ==
  data: x1 input single; y output single; x2 input single; r input single; h input single
function y = fhan(x1, x2, r, h)
    d = r * h^2;
    a0 = h * x2;
    y = x1 + a0;
    a1 = sqrt( d * (d + 8*abs(y)) );
    a2 = a0 + sign(y)*(a1 - d)/2;
    sy = (sign(y + d) - sign(y - d))/2;
    a = (a0 + y - a2)*sy + a2;
    sa = (sign(a + d) - sign(a - d))/2;
    y = -r*(a/d - sign(a))*sa - r*sign(a);

== matlab function AttitudeControl_ADRC_Sim/Control System/AttitudeControl/TD1/TD ==
  data: v input; v1_ output; r input; h input; v2_ output
function [v1_, v2_] = TD(v, r, h)
persistent v1 v2
if isempty(v1) || isempty(v2)
    v1 = 0;
    v2 = 0;
end

fv = fhan(v1 - v, v2, r,  h);
v1_ = v1 + h*v2;
v2_ = v2 + h*fv;

v1 = v1_;
v2 = v2_;
end

function y = fhan(x1, x2, r0, h0)

d = r0*h0^2;
a0 = h0*x2;
y = x1 + a0;
a1 = sqrt(d*(d + 8*abs(y)));
a2 = a0 + sign(y)*(a1 - d)/2;
sy = (sign(y + d) - sign(y - d))/2;%fsg
a = (a0 + y -a2)*sy + a2;
sa = (sign(a + d) - sign(a - d))/2;
y = -r0*(a/d - sign(a))*sa - r0*sign(a);

end

== matlab function AttitudeControl_ADRC_Sim/Quadcopter Dynamics/Rigid Model/Rigid-Body Kinematic Model /Quaternion to rotation matrix ==
  data: q input; Reb output
function Reb = fcn(q)
%Function description;
%  The rotation matrix of the Aircraft-Body Coordinate Frame (ABCF) to the
%  Earth-Fixed Coordinate Frame (EFCF) is obtained from the quaternions
Reb = [q(1)*q(1) + q(2)*q(2) - q(3)*q(3) - q(4)*q(4), 2*(q(2)*q(3) - q(1)*q(4)), 2*(q(2)*q(4) + q(1)*q(3))
           2*(q(2)*q(3) + q(1)*q(4)), q(1)*q(1) - q(2)*q(2) + q(3)*q(3) - q(4)*q(4), 2*(q(3)*q(4) - q(1)*q(2))
           2*(q(2)*q(4) - q(1)*q(3)), 2*(q(3)*q(4) + q(1)*q(2)), q(1)*q(1) - q(2)*q(2) - q(3)*q(3) + q(4)*q(4)];

== matlab function AttitudeControl_ADRC_Sim/Quadcopter Dynamics/Rigid Model/Rigid-Body Kinematic Model /Quaternion to Euler ==
  data: q input; y output
function y = fcn(q)
 %Function description:
%  Quaternions to Euler
phi = atan2(2*(q(1)*q(2) + q(3)*q(4)), (1 - 2*(q(2)*q(2) + q(3)*q(3))));
theta = asin(2*(q(1)*q(3) - q(2)*q(4)));
psi = atan2(2*(q(1)*q(4) + q(2)*q(3)), (1 - 2*(q(3)*q(3) + q(4)*q(4))));
y = [phi theta psi];

== matlab function AttitudeControl_ADRC_Sim/Quadcopter Dynamics/Rigid Model/Rigid-Body Kinematic Model /Quaternions model ==
  data: pqr input; qdot output; q input
function qdot = fcn(pqr, q)
%Function description:
%  Quaternions model
qdot = 0.5*[0, -pqr(1), -pqr(2), -pqr(3); pqr(1), 0, pqr(3), -pqr(2); pqr(2), -pqr(3), 0, pqr(1); pqr(3), pqr(2), -pqr(1), 0]*q;

== matlab function AttitudeControl_ADRC_Sim/Quadcopter Dynamics/Rigid Model/Rigid-Body Kinematic Model /Euler angle to quaternion ==
  data: EulerAngle input; q output
function q = fcn(EulerAngle)
%Function description:
%  Get quaternions from Euler angle
q0 =  cos(EulerAngle(1)/2)*cos(EulerAngle(2)/2)*cos(EulerAngle(3)/2) + sin(EulerAngle(1)/2)*sin((EulerAngle(2)/2))*sin((EulerAngle(3)/2));
q1 = sin(EulerAngle(1)/2)*cos(EulerAngle(2)/2)*cos(EulerAngle(3)/2) - cos(EulerAngle(1)/2)*sin((EulerAngle(2)/2))*sin((EulerAngle(3)/2));
q2 = cos(EulerAngle(1)/2)*sin(EulerAngle(2)/2)*cos(EulerAngle(3)/2) + sin(EulerAngle(1)/2)*cos((EulerAngle(2)/2))*sin((EulerAngle(3)/2));
q3 = cos(EulerAngle(1)/2)*cos(EulerAngle(2)/2)*sin(EulerAngle(3)/2) - sin(EulerAngle(1)/2)*sin((EulerAngle(2)/2))*cos((EulerAngle(3)/2));
q = [q0 q1 q2 q3]';

== matlab function AttitudeControl_ADRC_Sim/Quadcopter Dynamics/Control Effectiveness Model/Propeller Model ==
  data: w input; R input; Fp output; Fd output; Mp output; Cm input; Ct input; Vb input; Cd input; wb input; Md output; Cdm input; Jrp input; Ga output
function [Fp, Fd, Mp, Md, Ga] = fcn(w, R, Cm, Ct, Vb, Cd,wb, Cdm, Jrp)
 %Function description:
 %  Obtain the force and torque acting on the body. The airframe of the
 %  quadrotor is as follows:
 %3↓   1↑
 %  \ /
 %  / \
 %2↑   4↓
 %↑ stands for counterclockwise and ↓stands for clockwise.
 %Input：
 %  w: motor speed，unit：rad/s
 %  R: body radius(m)
 %  Cm: torque coefficient
 %  Ct: thrust coefficient
 %  Vb: aircraft speed in the body coordinate system
 %  Cd: damping coefficient
 %  wb: angular velocity in the body coordinate system
 %  Cdm: damping moment coefficient vector
 %  Jrp:  moment of inertia of motor rotor + propeller
 %Output:
 %  Fp: thrust under the body coordinate system
 %  Fd: aerodynamic force under the body coordinate system
 %  Mp: torque under the body coordinate system
 %  Md: aerodynamic moment
 %  Ga: gyro moment
 M_rctcm = [-sin(pi/4)*R*Ct, sin(pi/4)*R*Ct, sin(pi/4)*R*Ct, -sin(pi/4)*R*Ct;
            sin(pi/4)*R*Ct, -sin(pi/4)*R*Ct, sin(pi/4)*R*Ct, -sin(pi/4)*R*Ct;
            Cm, Cm, -Cm, -Cm];
 Mp = M_rctcm*(w.^2);  % torque
 
 Fp = [0; 0; -sum(Ct*(w.^2))];  % thrust
 Fd = -Cd*Vb.*abs(Vb)*0.5;  % aerodynamic force
 Md = -Cdm.*wb.*abs(wb);  % aerodynamic moment
 % gyro moment
 Ga = zeros(3,1);
 Ga(1) = Jrp*wb(2)*( w(1) + w(2) - w(3) - w(4));
 Ga(2) = Jrp*wb(1)*(-w(1) - w(2) + w(3) + w(4));
end

== matlab function AttitudeControl_ADRC_Sim/Control System/pwm_out2 ==
  data: Roll input; M1 output; Pitch input; Yaw input; Thrust input; M2 output; M3 output; M4 output
function [M1, M2, M3, M4] = motor_mixer(Roll, Pitch, Yaw, Thrust)
%Function description:
%  Control allocation. The quadrotor type is X-configuration,
%  and the airframe is as follows:
%3↓   1↑
 %  \ /
 %  / \
 %2↑   4↓
%Input：
%  Roll, Pitch, Yaw: attitude controller output.
%  Thrust

idle_PWM = 0;
scale = 1;

M1 = (Thrust - Roll + Pitch + Yaw) * scale + idle_PWM;
M2 = (Thrust + Roll - Pitch + Yaw) * scale + idle_PWM;
M3 = (Thrust + Roll + Pitch - Yaw) * scale + idle_PWM;
M4 = (Thrust - Roll - Pitch - Yaw) * scale + idle_PWM;
if M1 < 0
    M1 = single(0);
elseif M1 > 1
    M1 = single(1);  
end
if M2 < 0
    M2 = single(0);
elseif M2 > 1
    M2 = single(1);  
end
if M3<0
    M3 = single(0);
elseif M3 > 1
    M3 = single(1);  
end
if M4<0
    M4 = single(0);
elseif M4 > 1
    M4 = single(1);  
end

== matlab function AttitudeControl_ADRC_Sim/Control System/AttitudeControl/NLSEF/fhan ==
  data: x1 input single; y output single; x2 input single; r input single; h input single
function y = fhan(x1, x2, r, h)
    d = r * h^2;
    a0 = h * x2;
    y = x1 + a0;
    a1 = sqrt( d * (d + 8*abs(y)) );
    a2 = a0 + sign(y)*(a1 - d)/2;
    sy = (sign(y + d) - sign(y - d))/2;
    a = (a0 + y - a2)*sy + a2;
    sa = (sign(a + d) - sign(a - d))/2;
    y = -r*(a/d - sign(a))*sa - r*sign(a);

== matlab function AttitudeControl_ADRC_Sim/Control System/AttitudeControl/TD/TD ==
  data: v input; v1_ output; r input; h input; v2_ output
function [v1_, v2_] = TD(v, r, h)
persistent v1 v2
if isempty(v1) || isempty(v2)
    v1 = 0;
    v2 = 0;
end

fv = fhan(v1 - v, v2, r,  h);
v1_ = v1 + h*v2;
v2_ = v2 + h*fv;

v1 = v1_;
v2 = v2_;
end

function y = fhan(x1, x2, r0, h0)

d = r0*h0^2;
a0 = h0*x2;
y = x1 + a0;
a1 = sqrt(d*(d + 8*abs(y)));
a2 = a0 + sign(y)*(a1 - d)/2;
sy = (sign(y + d) - sign(y - d))/2;%fsg
a = (a0 + y -a2)*sy + a2;
sa = (sign(a + d) - sign(a - d))/2;
y = -r0*(a/d - sign(a))*sa - r0*sign(a);

end

== matlab function AttitudeControl_ADRC_Sim/Control System/AttitudeControl/ESO/adrc_eso ==
  settings: updateMethod=DISCRETE
  data: y input; u input; z1_ output; b01 input; b02 input; b03 input; b0 input; d input; h input; z2_ output; z3_ output
function [z1_, z2_, z3_] = adrc_eso(y, u, b01, b02, b03, b0, d, h)
persistent z1  z2 z3
if (isempty(z1) || isempty(z2) || isempty(z3))
    z1 = 0;
    z2 = 0;
    z3 = 0;
end
e = z1 - y;
fe = fal(e, 0.5, d);
fe1 = fal(e, 0.25, d);

z1_ = z1 + h*(z2 - b01*e);
z2_ = z2 + h*(z3 + b0*u - b02*fe);
z3_ = z3 - h*b03*fe1;

z1 = z1_;
z2 = z2_;
z3 = z3_;

end

function  y = fal( x, alpha, delta )

if abs(x) < delta
    y = x / delta^(1.0 - alpha);
else
    y = (abs(x)^alpha) * sign(x);
end

end

== matlab function AttitudeControl_ADRC_Sim/Control System/InputConditioning/f1 ==
  data: in input; y output; hover input
function y = thr_curve(in, hover)
%Function description:
%  After this function, when the throttle is in the middle position, the output is hovering throttle hover
%Input:
%  in: Throttle normalized value, range (0~1)
%  hover: Hovering throttle value
%Output:
%  Processed throttle value
if in < 0.5
	y=2 * in * hover;
else
	y=hover + 2 * (in - 0.5) * (1.0 - hover);
end
